simulink model "example_House_Simple_ISO_GroundModel"  (R2013b)
settings: Solver=ode45  StartTime=0.0  StopTime=10*24*3600  RelTol=1e-3
libraries: carnot x4
settings Model: Creator=drhf  LastModifiedBy=drhf
settings SolverCC: ZeroCrossAlgorithm=Adaptive
settings OptimizationCC: ExpressionDepthLimit=2147483647
settings DebuggingCC: StateNameClashWarn=warning
settings GRTTargetCC: CombineOutputUpdateFcns=off  GRTInterface=on

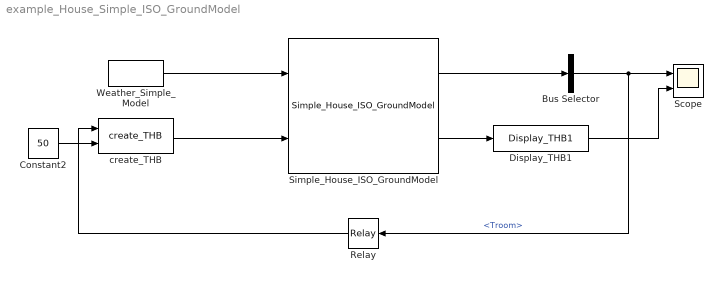
== system example_House_Simple_ISO_GroundModel ==
  Bus Selector : BusSelector  OutputSignals=Troom
  Constant2 : Constant  Value=50
  Display_THB1 : carnot/Outputs/Display_THB1  t=off  m=on  p=off  id=off  mix=off  d=off
  Relay : Relay  OnSwitchValue=20.1  OffSwitchValue=19.9  OnOutputValue=0  OffOutputValue=720/3600
  Scope : Scope  NumInputPorts=2
      settings: YMin=-5~-5  YMax=5~5
  Simple_House_ISO_GroundModel : carnot/Load/Houses/Simple_House_ISO_GroundModel  Ahabit=140  Hroom=2.6  Floorsize=[7 10]  UAwall=0.5*(54.6+26.4)+0.182*((45.7+56.0)*2 -(12+4+3+4))  UAneighbour=0  Uground=0.2  mc=0.5e6*140 % 0.5 MJ/m2/K  Awin=[12 4 3 4]  AziWin=[0 90 -180 -90]  Uwin="[1    1   1    1]*2.0"  Gwin="[1    1   1    1]*0.585*(1-0.15)"  shade=0.75  tini=20  vent=0.4  rec=0.6  uaheating=425 %400  dpcoeff=[10 100]  heatload=1792  delta_t_nom=15  n_rad=1.1  mass_times_cap=40e6
  Weather_Simple_Model : carnot/Weather/Weather_Simple_Model  lat=60  Ibn=900  Idg=100  tamb=5  deltaTsky=-6  rh=50  precip="10e-3/24/3600           % 10 mm in 24 h"  cloud=0.125  p=1013e2  vw=1  wdir=270
  create_THB : carnot/Source/Simple/create_THB  p=1e5  fluid=Water  mix=0  dia=0.02  mID=No Pressure Drop
  wires:
  Bus Selector/1 -> Scope/1, Relay/1  "<Troom>"
  Constant2/1 -> create_THB/2
  Relay/1 -> create_THB/1
  Weather_Simple_Model/1 -> Simple_House_ISO_GroundModel/1
  create_THB/1 -> Simple_House_ISO_GroundModel/2
  Simple_House_ISO_GroundModel/1 -> Bus Selector/1
  Simple_House_ISO_GroundModel/2 -> Display_THB1/1
  Display_THB1/1 -> Scope/2
